simulink model "ModelAgriAuto"  (R2022a)
settings: Solver=FixedStepAuto  StartTime=0.0  StopTime=6240  FixedStep=0.05  MaxStep=0.1  RelTol=1e-3
model workspace (MAT data in the model file):
  PlowHectare = 1.925
values from neighbouring files (symbols this model uses):
  C_rate = 3    [start_function.m]
  Compaction = 0    [start_function.m]
  CyclesIn = CyclesIn+CyclesOut(end)    [start_function.m]
  Degradation = 2    [start_function.m]
  FailRate = 29700000    [start_function.m]
  FieldEff = 0.8    [start_function.m]
  ForceCorrVar = 0.85    [start_function.m]
  Fuel = 3    [start_function.m]
  Mass = 10550    [start_function.m]
  n = n+1    (= 2)    [start_function.m]
  v_field = 5    [start_function.m]
  Weather_crit = 3    [start_function.m]
  WorkingHours = 10    [start_function.m]
undefined symbols (not defined in the file or in its folder): Battery, BatteryNo, Charger, ChargerNo, DField, m, Power, Soil, TractorNo, Year
libraries: simulink x2
(part 2 of 3)

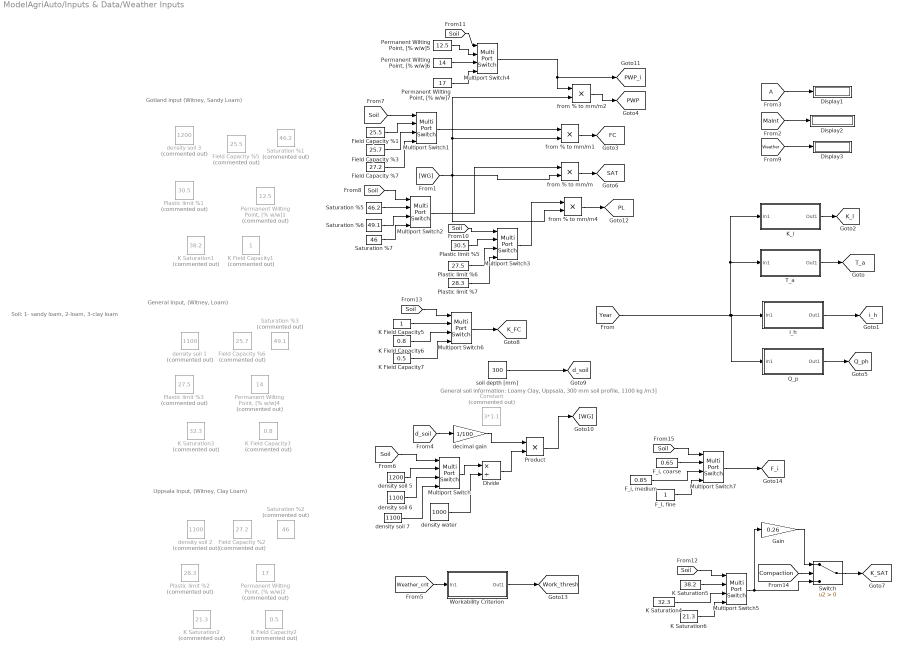
== system ModelAgriAuto/Inputs & Data/Weather Inputs ==
  note: Soil: 1- sandy loam, 2-loam, 3-clay loam
  note: Uppsala Input, (Witney, Clay Loam)
  note: Gotland input (Witney, Sandy Loam)
  note: General soil information: Loamy Clay, Uppsala, 300 mm soil profile, 1100 kg /m3]
  note: General Input, (Witney, Loam)
  Constant : Constant  Commented=on  Value=3*1.1
  Display1 : Display
  Display2 : Display
  Display3 : Display
  Divide : Product  Inputs=*/
  "F_I, fine" : Constant
  "F_i, coarse" : Constant  Value=0.65
  "F_i, medium" : Constant  Value=0.85
  Field Capacity %1 : Constant  Value=25.5
  Field Capacity %2 : Constant  Commented=on  Value=27.2
  Field Capacity %3 : Constant  Value=25.7
  Field Capacity %5 : Constant  Commented=on  Value=25.5
  Field Capacity %6 : Constant  Commented=on  Value=25.7
  Field Capacity %7 : Constant  Value=27.2
  From3 : From  TagVisibility=global
  Gain : Gain  Gain=0.26
  K Field Capacity1 : Constant  Commented=on
  K Field Capacity2 : Constant  Commented=on  Value=0.5
  K Field Capacity3 : Constant  Commented=on  Value=0.8
  K Field Capacity5 : Constant
  K Field Capacity6 : Constant  Value=0.8
  K Field Capacity7 : Constant  Value=0.5
  K Saturation1 : Constant  Commented=on  Value=38.2
  K Saturation2 : Constant  Commented=on  Value=21.3
  K Saturation3 : Constant  Commented=on  Value=32.3
  K Saturation4 : Constant  Value=32.3
  K Saturation5 : Constant  Value=38.2
  K Saturation6 : Constant  Value=21.3
  K_l : Subsystem
  Multiport Switch{,1..7} (8 alike) : MultiPortSwitch  SaturateOnIntegerOverflow=off  InputSameDT=off
  "Permanent Wilting Point, [% w/w]1" : Constant  Commented=on  Value=12.5
  "Permanent Wilting Point, [% w/w]2" : Constant  Commented=on  Value=17
  "Permanent Wilting Point, [% w/w]4" : Constant  Commented=on  Value=14
  "Permanent Wilting Point, [% w/w]5" : Constant  Value=12.5
  "Permanent Wilting Point, [% w/w]6" : Constant  Value=14
  "Permanent Wilting Point, [% w/w]7" : Constant  Value=17
  Plastic limit %1 : Constant  Commented=on  Value=30.5
  Plastic limit %2 : Constant  Commented=on  Value=28.3
  Plastic limit %3 : Constant  Commented=on  Value=27.5
  Plastic limit %5 : Constant  Value=30.5
  Plastic limit %6 : Constant  Value=27.5
  Plastic limit %7 : Constant  Value=28.3
  Product : Product
  Q_p : Subsystem
  Saturation %1 : Constant  Commented=on  Value=46.2
  Saturation %2 : Constant  Commented=on  Value=46
  Saturation %3 : Constant  Commented=on  Value=49.1
  Saturation %5 : Constant  Value=46.2
  Saturation %6 : Constant  Value=49.1
  Saturation %7 : Constant  Value=46
  Switch : Switch  Criteria=u2 > Threshold  SaturateOnIntegerOverflow=off  InputSameDT=off
  T_a : Subsystem
  "Workability Criterion " : Subsystem
  decimal gain : Gain  Gain=1/100
  density soil 1 : Constant  Commented=on  Value=1100
  density soil 2 : Constant  Commented=on  Value=1100
  density soil 3 : Constant  Commented=on  Value=1200
  density soil 5 : Constant  Value=1200
  density soil 6 : Constant  Value=1100
  density soil 7 : Constant  Value=1100
  "density water " : Constant  Value=1000
  from % to mm/m{,1..2,4} (4 alike) : Product
  i_h : Subsystem
  soil depth [mm] : Constant  Value=300
  tag scope: FC=global, F_i=global, K_FC=global, K_SAT=global, K_l=global, PL=global, PWP=global, PWP_i=global, Q_ph=global, SAT=global, T_a=global, Work_thresh=global, d_soil=global, i_h=global
  wires:
  K_l/1(Out1) -> [K_l]
  T_a/1(Out1) -> [T_a]
  i_h/1(Out1) -> [i_h]
  Q_p/1(Out1) -> [Q_ph]
  From3/1 -> Display1/1
  [Weather] -> Display3/1
  [MaInt] -> Display2/1
  Multiport Switch4/1 -> from % to mm/m2/1, [PWP_i]
  Multiport Switch2/1 -> from % to mm/m/1
  Multiport Switch6/1 -> [K_FC]
  soil depth [mm]/1 -> [d_soil]
  [WG] -> from % to mm/m4/2, from % to mm/m2/2, from % to mm/m1/2, from % to mm/m/2
  from % to mm/m/1 -> [SAT]
  from % to mm/m1/1 -> [FC]
  from % to mm/m2/1 -> [PWP]
  Divide/1 -> Product/2
  [d_soil] -> decimal gain/1
  "density water "/1 -> Divide/2
  decimal gain/1 -> Product/1
  Product/1 -> [WG]
  Multiport Switch3/1 -> from % to mm/m4/1
  from % to mm/m4/1 -> [PL]
  Multiport Switch/1 -> Divide/1
  Multiport Switch1/1 -> from % to mm/m1/1
  [Soil] -> Multiport Switch/1
  density soil 5/1 -> Multiport Switch/2
  density soil 6/1 -> Multiport Switch/3
  density soil 7/1 -> Multiport Switch/4
  [Soil] -> Multiport Switch1/1
  Field Capacity %7/1 -> Multiport Switch1/4
  Field Capacity %1/1 -> Multiport Switch1/2
  Field Capacity %3/1 -> Multiport Switch1/3
  Saturation %7/1 -> Multiport Switch2/4
  [Soil] -> Multiport Switch2/1
  Saturation %5/1 -> Multiport Switch2/2
  Saturation %6/1 -> Multiport Switch2/3
  [Soil] -> Multiport Switch3/1
  Plastic limit %5/1 -> Multiport Switch3/2
  Plastic limit %6/1 -> Multiport Switch3/3
  Plastic limit %7/1 -> Multiport Switch3/4
  "Workability Criterion "/1(Out1) -> [Work_thresh]
  [Weather_crit] -> "Workability Criterion "/1(In1)
  "Permanent Wilting Point, [% w/w]6"/1 -> Multiport Switch4/3
  [Soil] -> Multiport Switch4/1
  "Permanent Wilting Point, [% w/w]5"/1 -> Multiport Switch4/2
  "Permanent Wilting Point, [% w/w]7"/1 -> Multiport Switch4/4
  K Saturation4/1 -> Multiport Switch5/3
  [Soil] -> Multiport Switch5/1
  K Saturation6/1 -> Multiport Switch5/4
  K Saturation5/1 -> Multiport Switch5/2
  K Field Capacity7/1 -> Multiport Switch6/4
  [Soil] -> Multiport Switch6/1
  K Field Capacity5/1 -> Multiport Switch6/2
  K Field Capacity6/1 -> Multiport Switch6/3
  [Compaction] -> Switch/2
  Multiport Switch5/1 -> Gain/1, Switch/3
  Switch/1 -> [K_SAT]
  Gain/1 -> Switch/1
  "F_I, fine"/1 -> Multiport Switch7/4
  "F_i, medium"/1 -> Multiport Switch7/3
  "F_i, coarse"/1 -> Multiport Switch7/2
  [Soil] -> Multiport Switch7/1
  Multiport Switch7/1 -> [F_i]
  [Year] -> K_l/1(In1), T_a/1(In1), Q_p/1(In1), i_h/1(In1)

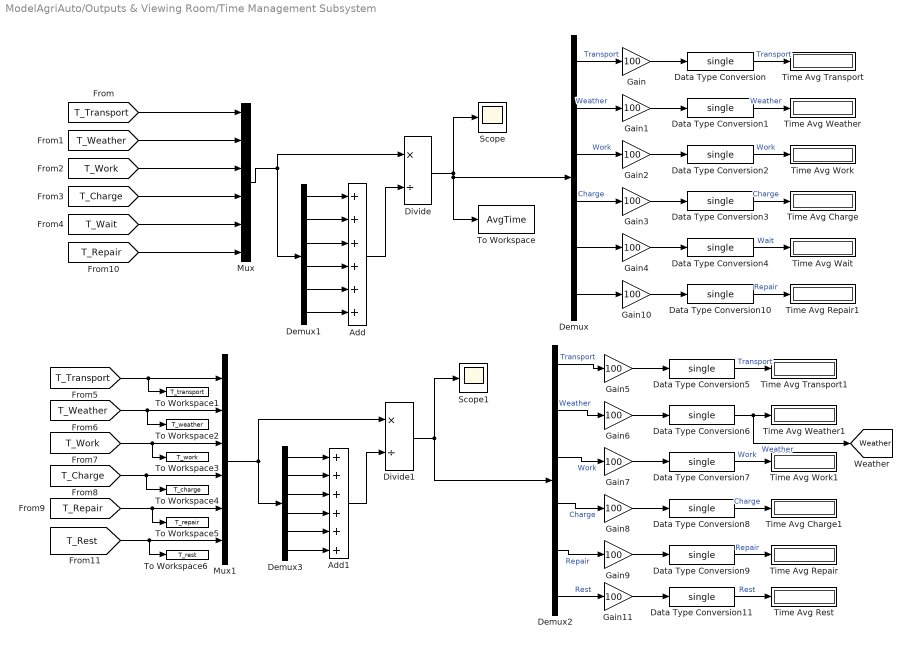
== system ModelAgriAuto/Outputs & Viewing Room/Time Management Subsystem ==
  Add : Sum  Inputs=++++++
  Add1 : Sum  Inputs=++++++
  Data Type Conversion{,1..11} (12 alike) : DataTypeConversion  OutDataTypeStr=single  SaturateOnIntegerOverflow=off  RndMeth=Floor
  Demux{,1..3} (4 alike) : Demux  Outputs=6
  Divide : Product  Inputs=*/
  Divide1 : Product  Inputs=*/
  Gain{,1..11} (12 alike) : Gain  Gain=100
  Mux : Mux  Inputs=6
  Mux1 : Mux  Inputs=6
  Scope : Scope
  Scope1 : Scope
  Time Avg Charge : Display
  Time Avg Charge1 : Display
  Time Avg Repair : Display
  Time Avg Repair1 : Display
  Time Avg Rest : Display
  Time Avg Transport : Display
  Time Avg Transport1 : Display
  Time Avg Wait : Display
  Time Avg Weather : Display
  Time Avg Weather1 : Display
  Time Avg Work : Display
  Time Avg Work1 : Display
  To Workspace : ToWorkspace  VariableName=AvgTime  SaveFormat=Timeseries  SampleTime=1
  To Workspace1 : ToWorkspace  VariableName=T_transport  SampleTime=1
      settings: Save2DSignal=2-D array (concatenate along first dimension)
  To Workspace2 : ToWorkspace  VariableName=T_weather  SampleTime=1
      settings: Save2DSignal=2-D array (concatenate along first dimension)
  To Workspace3 : ToWorkspace  VariableName=T_work  SampleTime=1
      settings: Save2DSignal=2-D array (concatenate along first dimension)
  To Workspace4 : ToWorkspace  VariableName=T_charge  SampleTime=1
      settings: Save2DSignal=2-D array (concatenate along first dimension)
  To Workspace5 : ToWorkspace  VariableName=T_repair  SampleTime=1
      settings: Save2DSignal=2-D array (concatenate along first dimension)
  To Workspace6 : ToWorkspace  VariableName=T_rest  SampleTime=1
      settings: Save2DSignal=2-D array (concatenate along first dimension)
  tag scope: Weather=global
  wires:
  [T_Transport] -> Mux/1
  [T_Weather] -> Mux/2
  [T_Work] -> Mux/3
  [T_Charge] -> Mux/4
  Mux/1 -> Divide/1, Demux1/1
  Divide/1 -> Demux/1, To Workspace/1, Scope/1
  Demux/1 -> Gain/1  "Transport"
  Demux/2 -> Gain1/1  "Weather"
  Demux/3 -> Gain2/1  "Work"
  Demux/4 -> Gain3/1  "Charge"
  Demux1/2 -> Add/2
  Demux1/1 -> Add/1
  Demux1/3 -> Add/3
  Demux1/4 -> Add/4
  Add/1 -> Divide/2
  Data Type Conversion/1 -> Time Avg Transport/1  "Transport"
  Data Type Conversion1/1 -> Time Avg Weather/1  "Weather"
  Data Type Conversion2/1 -> Time Avg Work/1  "Work"
  Data Type Conversion3/1 -> Time Avg Charge/1  "Charge"
  Gain/1 -> Data Type Conversion/1
  Gain1/1 -> Data Type Conversion1/1
  Gain2/1 -> Data Type Conversion2/1
  Gain3/1 -> Data Type Conversion3/1
  [T_Wait] -> Mux/5
  Demux1/5 -> Add/5
  Demux/5 -> Gain4/1
  Gain4/1 -> Data Type Conversion4/1
  Data Type Conversion4/1 -> Time Avg Wait/1  "Wait"
  Data Type Conversion5/1 -> Time Avg Transport1/1  "Transport"
  Mux1/1 -> Divide1/1, Demux3/1
  Demux2/3 -> Gain7/1  "Work"
  Demux2/1 -> Gain5/1  "Transport"
  [T_Charge] -> To Workspace4/1, Mux1/4
  Demux3/4 -> Add1/4
  Add1/1 -> Divide1/2
  Gain6/1 -> Data Type Conversion6/1
  Demux3/3 -> Add1/3
  Gain5/1 -> Data Type Conversion5/1
  [T_Work] -> To Workspace3/1, Mux1/3
  Demux2/4 -> Gain8/1  "Charge"
  [T_Transport] -> To Workspace1/1, Mux1/1
  Gain8/1 -> Data Type Conversion8/1
  Gain7/1 -> Data Type Conversion7/1
  Divide1/1 -> Scope1/1, Demux2/1
  Data Type Conversion6/1 -> [Weather], Time Avg Weather1/1  "Weather"
  [T_Weather] -> To Workspace2/1, Mux1/2
  Demux3/1 -> Add1/1
  Data Type Conversion7/1 -> Time Avg Work1/1  "Work"
  Data Type Conversion8/1 -> Time Avg Charge1/1  "Charge"
  Demux2/2 -> Gain6/1  "Weather"
  Demux3/2 -> Add1/2
  [T_Repair] -> To Workspace5/1, Mux1/5
  Demux3/5 -> Add1/5
  Demux2/5 -> Gain9/1  "Repair"
  Gain9/1 -> Data Type Conversion9/1
  Data Type Conversion9/1 -> Time Avg Repair/1  "Repair"
  [T_Repair] -> Mux/6
  Demux1/6 -> Add/6
  Gain10/1 -> Data Type Conversion10/1
  Data Type Conversion10/1 -> Time Avg Repair1/1  "Repair"
  Demux/6 -> Gain10/1
  [T_Rest] -> To Workspace6/1, Mux1/6
  Demux3/6 -> Add1/6
  Gain11/1 -> Data Type Conversion11/1
  Data Type Conversion11/1 -> Time Avg Rest/1  "Rest"
  Demux2/6 -> Gain11/1  "Rest"

== system ModelAgriAuto/Time & Weather subsyst./Driver work-time subsystem ==
  note: Working time check
  In1 : Inport
  Add : Sum  Inputs=+-
  Avg wait time [h]1 : Display
  Constant : Constant  Value=0
  Constant1 : Constant
  Counter Limited : simulink/Sources/Counter Limited  uplimit=24  tsamp=1
  Entity Gate : EntityGate  InputPortMessageModes=m,m  OutputPortMessageModes=m  OpenGateAtSimulationStart=on
  Entity Queue2 : Queue  InputPortMessageModes=m  OutputPortMessageModes=n,n,m  NumberEntitiesDeparted=on  AverageWait=on
      settings: OutputPortMap=o0,o2,o5
  Message Send1 : Send  OutputPortMessageModes=m
  Product : Product
  Switch : Switch  SaturateOnIntegerOverflow=off  InputSameDT=off
  Out1 : Outport
  tag scope: T_Rest=global
  wires:
  Add/1 -> Switch/2
  [WorkingHours] -> Add/2
  Constant/1 -> Switch/1
  Constant1/1 -> Switch/3
  Counter Limited/1 -> Add/1
  In1/1 -> Entity Queue2/1
  Entity Queue2/3 -> Entity Gate/2
  Entity Gate/1 -> Out1/1
  Message Send1/1 -> Entity Gate/1
  Switch/1 -> Message Send1/1
  Entity Queue2/1 -> Product/2
  Entity Queue2/2 -> Product/1
  Product/1 -> Avg wait time [h]1/1, [T_Rest]

== system ModelAgriAuto/Time & Weather subsyst./Weather & schedule subsystem ==
  note: From Alfredo (2004)
  note: Working time check
  note: Soil moisture check
  In1 : Inport
  % of days workable : Display
  Add : Sum  Inputs=+-
  Avg wait time [h]1 : Display
  Clock1 : Clock
  Constant : Constant  Value=0
  Constant1 : Constant
  Counter Limited : simulink/Sources/Counter Limited  uplimit=24  tsamp=1
  "Daily soil water content model " : Subsystem
  Divide1 : Product  Inputs=*/
  Entity Gate : EntityGate  InputPortMessageModes=m,m  OutputPortMessageModes=m  OpenGateAtSimulationStart=on
  Entity Queue2 : Queue  InputPortMessageModes=m  OutputPortMessageModes=n,n,m  NumberEntitiesDeparted=on  AverageWait=on
      settings: OutputPortMap=o0,o2,o5
  Gain : Gain  Gain=100
  Integrator : Integrator
  Integrator1 : Integrator
  Message Send1 : Send  OutputPortMessageModes=m
  Product : Product
  Product1 : Product
  Relational Operator1 : RelationalOperator  Operator=<=  OutDataTypeStr='double'  InputSameDT=off
  Scope : Scope
  Scope1 : Scope  NumInputPorts=2
  Switch : Switch  SaturateOnIntegerOverflow=off  InputSameDT=off
  Threshold value (mm/m) : Display
  To Workspace : ToWorkspace  VariableName=WeatherWaitTime1  SaveFormat=Timeseries  SampleTime=1
  To Workspace1 : ToWorkspace  VariableName=m_a1  SampleTime=1
  Utilization : Scope
  Workable : Goto  TagVisibility=global
  Out1 : Outport  VectorParamsAs1DForOutWhenUnconnected=off
  tag scope: MaInt=global, T_Weather=global, Workability=global
  wires:
  Entity Queue2/3 -> Entity Gate/2
  Clock1/1 -> Divide1/2
  [Work_thresh] -> Relational Operator1/2, Threshold value (mm/m)/1
  Entity Gate/1 -> Out1/1
  Entity Queue2/1 -> Product/2
  Divide1/1 -> Workable/1, Gain/1
  Relational Operator1/1 -> Scope1/1, Product1/1, [Workability], Utilization/1, Integrator1/1
  Gain/1 -> % of days workable/1
  Switch/1 -> Scope1/2, Product1/2
  Message Send1/1 -> Entity Gate/1
  Entity Queue2/2 -> Avg wait time [h]1/1, Product/1
  Integrator/1 -> [MaInt]
  Integrator1/1 -> Divide1/1
  Add/1 -> Switch/2
  [WorkingHours] -> Add/2
  "Daily soil water content model "/1(m_a (Soil moisture content [mm/m])) -> Integrator/1, To Workspace1/1, Relational Operator1/1
  In1/1 -> Entity Queue2/1
  Constant/1 -> Switch/1
  Product1/1 -> Scope/1, Message Send1/1
  Constant1/1 -> Switch/3
  Counter Limited/1 -> Add/1
  Product/1 -> [T_Weather], To Workspace/1

== system ModelAgriAuto/Transport Subsystem/Road forces ==
  "m " : Inport
  a : Inport  Port=2
  "N_block " : Inport  Port=3
  *g : Gain  Gain=9.81
  Crr_road : Constant  Value=0.1
  Display : Display
  Drag force road : MATLAB Function  TreatAsAtomicUnit=on
  Integrator : Integrator
  "Net force needed [N] " : Sum
  P [kW] : Scope
  "P [kW] " : Product  Inputs=3
  "Rolling resistance road " : Product
  Scope : Scope
  Subsystem : Subsystem
  "W to kW " : Constant  Value=0.001
  kWs to kWh : Gain  Gain=1/3600
  km/h to m/s : Gain  Gain=1/3.6
  tag scope: F_road=global, P_road=global, v_road=global
  wires:
  [v_road_actual] -> km/h to m/s/1, Drag force road/1(v)
  Drag force road/1(F_drag_road) -> "Net force needed [N] "/2
  a/1 -> Subsystem/1(a)
  "m "/1 -> *g/1
  Crr_road/1 -> "Rolling resistance road "/1
  *g/1 -> "Rolling resistance road "/2
  "Rolling resistance road "/1 -> "Net force needed [N] "/1
  "Net force needed [N] "/1 -> [F_road], "P [kW] "/1
  "W to kW "/1 -> "P [kW] "/3
  km/h to m/s/1 -> [v_road], "P [kW] "/2
  kWs to kWh/1 -> Scope/1
  "P [kW] "/1 -> Integrator/1, Display/1, [P_road], P [kW]/1
  Integrator/1 -> kWs to kWh/1
  "N_block "/1 -> Subsystem/2(In1)

== system ModelAgriAuto/Inputs & Data/Battery and driveline inputs/Battery capacity reduction ==
  Add : Sum  Inputs=++++
  Add1 : Sum
  Add2 : Sum
  Charging rate choice : Subsystem
  Constant4 : Constant  Value=BatteryNo
  Constant5 : Constant  Value=CyclesIn
  Constant7 : Constant  Value=TractorNo
  Constant8 : Constant  Value=0
  Display : Display
  Display1 : Display
  Display2 : Display
  Divide : Product  Inputs=*/
  Memory : Memory  InitialCondition=CyclesIn
  Product1 : Product  Inputs=3
  Product2 : Product
  Product4 : Product  Inputs=4
  Saturation : Saturate  UpperLimit=1
  Scope : Scope
  Switch : Switch  Criteria=u2 > Threshold  Threshold=1  SaturateOnIntegerOverflow=off  InputSameDT=off
  To Workspace : ToWorkspace  VariableName=CyclesOut  SampleTime=-1
      settings: Save2DSignal=2-D array (concatenate along first dimension)
  Out1 : Outport  VectorParamsAs1DForOutWhenUnconnected=off
  wires:
  Product1/1 -> Add/2
  Product2/1 -> Add/3
  Add/1 -> Saturation/1
  [Charge_no] -> Display1/1, Divide/1
  Saturation/1 -> Display2/1, Scope/1, Out1/1
  Product4/1 -> Add/1
  Memory/1 -> Display/1, Product4/4, Product4/2, Product4/3, Product1/2, Product1/3, Product2/1
  Constant4/1 -> Switch/1
  Divide/1 -> To Workspace/1, Add1/1
  Constant5/1 -> Add1/2
  Add1/1 -> Memory/1
  Constant7/1 -> Add2/2
  Add2/1 -> Divide/2
  Constant8/1 -> Switch/3
  Switch/1 -> Add2/1
  [Fuel] -> Switch/2
  Charging rate choice/1(Out1) -> Product4/1
  Charging rate choice/2(Out2) -> Product1/1
  Charging rate choice/3(Out3) -> Product2/2
  Charging rate choice/4(Out4) -> Add/4

== system ModelAgriAuto/Inputs & Data/Field inputs/Field efficiancy ==
  note: 0.8 From Witney
  Crop choice : MultiPortSwitch  Commented=on  Inputs=12  SaturateOnIntegerOverflow=off  InputSameDT=off
  Demux1 : Demux  Commented=on  Outputs=12
  Field effiency : Constant  Commented=on  Value=0.8  SampleTime=100000
  Field sizes [ha]1 : Constant  Commented=on  Value=[0.8 0.8 0.8 0.8 0.8 0.8 0.8 0.8 0.8 0.8 0.8 0.8]
  From2 : From  Commented=on  GotoTag=Field  TagVisibility=global
  Goto1 : Goto  Commented=on  GotoTag=field_eff  TagVisibility=global
  Goto4 : Goto  Commented=on  GotoTag=field_eff  TagVisibility=global
  wires:
  Field effiency/1 -> Goto4/1
  From2/1 -> Crop choice/1
  Demux1/5 -> Crop choice/6
  Demux1/6 -> Crop choice/7
  Demux1/9 -> Crop choice/10
  Demux1/7 -> Crop choice/8
  Demux1/3 -> Crop choice/4
  Demux1/2 -> Crop choice/3
  Demux1/8 -> Crop choice/9
  Demux1/12 -> Crop choice/13
  Demux1/4 -> Crop choice/5
  Demux1/10 -> Crop choice/11
  Demux1/11 -> Crop choice/12
  Demux1/1 -> Crop choice/2
  Field sizes [ha]1/1 -> Demux1/1
  Crop choice/1 -> Goto1/1

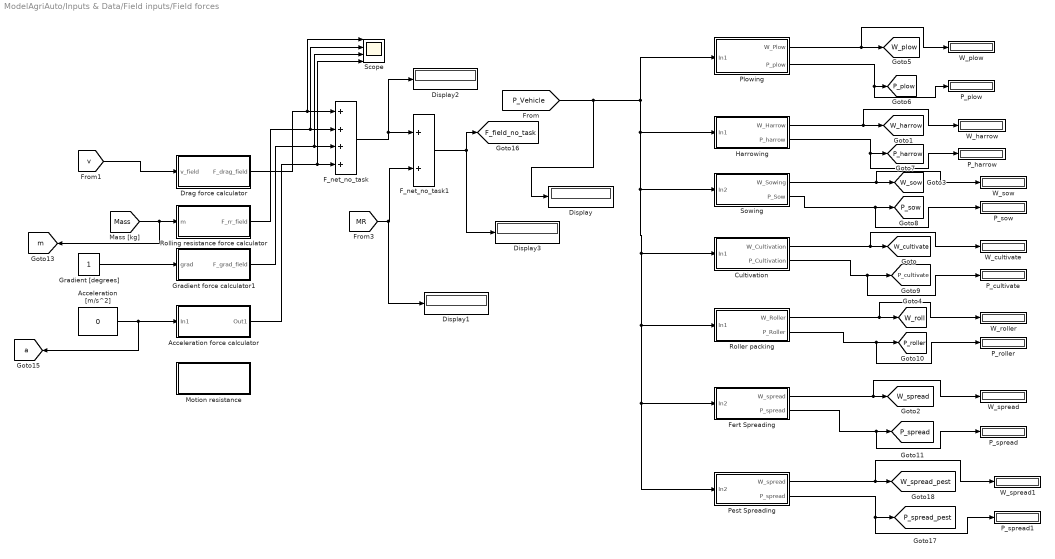
== system ModelAgriAuto/Inputs & Data/Field inputs/Field forces ==
  Acceleration [m/s^2] : Constant  Value=0
  Acceleration force calculator : Subsystem
  Cultivation : Subsystem
  Display{,1..3} (4 alike) : Display
  Drag force calculator : Subsystem
  F_net_no_task : Sum  Inputs=4
  F_net_no_task1 : Sum  Inputs=2
  Fert Spreading : Subsystem
  Gradient [degrees] : Constant
  Gradient force calculator1 : Subsystem
  Harrowing : Subsystem
  "Motion resistance " : Subsystem
  P_cultivate : Display
  P_harrow : Display
  P_plow : Display
  P_roller : Display
  P_sow : Display
  P_spread : Display
  P_spread1 : Display
  Pest Spreading : Subsystem
  Plowing : Subsystem
  Roller packing : Subsystem
  Rolling resistance force calculator : Subsystem
  Scope : Scope  NumInputPorts=4
  Sowing : Subsystem
  W_cultivate : Display
  W_harrow : Display
  W_plow : Display
  W_roller : Display
  W_sow : Display
  W_spread : Display
  W_spread1 : Display
  tag scope: F_field_no_task=global, P_cultivate=global, P_harrow=global, P_plow=global, P_roller=global, P_sow=global, P_spread=global, P_spread_pest=global, W_cultivate=global, W_harrow=global, W_plow=global, W_roll=global, W_sow=global, W_spread=global, W_spread_pest=global, a=global, m=global
  wires:
  Cultivation/1(W_Cultivation) -> W_cultivate/1, [W_cultivate]
  Roller packing/1(W_Roller) -> W_roller/1, [W_roll]
  Plowing/1(W_Plow) -> W_plow/1, [W_plow]
  Sowing/1(W_Sowing) -> W_sow/1, [W_sow]
  Harrowing/1(W_Harrow) -> W_harrow/1, [W_harrow]
  [P_Vehicle] -> Display/1, Sowing/1(In2), Cultivation/1(In1), Pest Spreading/1(In2), Fert Spreading/1(In2), Roller packing/1(In1), Harrowing/1(In1), Plowing/1(In1)
  Fert Spreading/1(W_spread) -> W_spread/1, [W_spread]
  Plowing/2(P_plow) -> P_plow/1, [P_plow]
  Harrowing/2(P_harrow) -> P_harrow/1, [P_harrow]
  Sowing/2(P_Sow) -> P_sow/1, [P_sow]
  Cultivation/2(P_Cultivation) -> P_cultivate/1, [P_cultivate]
  Roller packing/2(P_Roller) -> P_roller/1, [P_roller]
  Fert Spreading/2(P_spread) -> P_spread/1, [P_spread]
  F_net_no_task1/1 -> Display3/1, [F_field_no_task]
  [Mass] -> Rolling resistance force calculator/1(m), [m]
  Gradient [degrees]/1 -> Gradient force calculator1/1(grad)
  Rolling resistance force calculator/1(F_rr_field) -> Scope/2, F_net_no_task/2
  Acceleration force calculator/1(Out1) -> Scope/4, F_net_no_task/4
  Acceleration [m/s^2]/1 -> [a], Acceleration force calculator/1(In1)
  Drag force calculator/1(F_drag_field) -> Scope/1, F_net_no_task/1
  Pest Spreading/2(P_spread) -> P_spread1/1, [P_spread_pest]
  Pest Spreading/1(W_spread) -> W_spread1/1, [W_spread_pest]
  F_net_no_task/1 -> Display2/1, F_net_no_task1/1
  [MR] -> Display1/1, F_net_no_task1/2
  Gradient force calculator1/1(F_grad_field) -> Scope/3, F_net_no_task/3
  [v] -> Drag force calculator/1(v_field)

== system ModelAgriAuto/Inputs & Data/Field inputs/Fieldwork choice & data ==
  Crop choice : MultiPortSwitch  Inputs=12  SaturateOnIntegerOverflow=off  InputSameDT=off
  Demux : Demux  Outputs=16
  Demux1 : Demux  Outputs=12
  Fall period no. tasks : Constant  Value=8
  Havre / Oats : Subsystem
  Höstvete / Winter Wheat : Subsystem
  Korn / Barley : Subsystem
  Multiport Switch : MultiPortSwitch  Inputs=4  SaturateOnIntegerOverflow=off  InputSameDT=off
  Spring period no. tasks : Constant  Value=5
  Subsystem : Subsystem
  "Summer period no. tasks " : Constant  Value=3
  Task : MultiPortSwitch  Inputs=16  DiagnosticForDefault=None  SaturateOnIntegerOverflow=off  InputSameDT=off
  To Workspace : ToWorkspace  VariableName=P_vehicle  SampleTime=1
  To Workspace1 : ToWorkspace  VariableName=P_task  SampleTime=1
  To Workspace2 : ToWorkspace  VariableName=Task_no  SampleTime=1
  Vårvete / Spring wheat : Subsystem
  tag scope: P_fieldwork=global, W_fieldwork=global, X_1=global, X_2=global, X_3=global, X_val=global
  wires:
  Korn / Barley/1(Barley) -> Multiport Switch/3
  Havre / Oats/1(Oats) -> Multiport Switch/2
  Vårvete / Spring wheat/1(Spring Wheat) -> Multiport Switch/4
  Höstvete / Winter Wheat/1(Winter Wheat) -> Multiport Switch/5
  Subsystem/1(P) -> To Workspace1/1, [P_fieldwork]
  Subsystem/2(W) -> [W_fieldwork]
  Demux1/1 -> Crop choice/2
  Demux1/10 -> Crop choice/11
  Demux1/12 -> Crop choice/13
  Demux1/2 -> Crop choice/3
  Demux1/4 -> Crop choice/5
  Demux1/6 -> Crop choice/7
  [Rotation_choice] -> Demux1/1
  Demux1/11 -> Crop choice/12
  Demux1/3 -> Crop choice/4
  Demux1/9 -> Crop choice/10
  Demux1/7 -> Crop choice/8
  Demux1/8 -> Crop choice/9
  Demux1/5 -> Crop choice/6
  [Field] -> Crop choice/1
  Crop choice/1 -> Multiport Switch/1
  Spring period no. tasks/1 -> [X_1]
  "Summer period no. tasks "/1 -> [X_2]
  Fall period no. tasks/1 -> [X_3]
  Multiport Switch/1 -> Demux/1
  Task/1 -> [X_val], Subsystem/1(In1)
  Demux/1 -> Task/2
  Demux/2 -> Task/3
  Demux/3 -> Task/4
  Demux/4 -> Task/5
  Demux/5 -> Task/6
  Demux/6 -> Task/7
  Demux/7 -> Task/8
  Demux/8 -> Task/9
  Demux/9 -> Task/10
  Demux/10 -> Task/11
  Demux/11 -> Task/12
  Demux/12 -> Task/13
  Demux/13 -> Task/14
  Demux/14 -> Task/15
  Demux/15 -> Task/16
  Demux/16 -> Task/17
  [X] -> To Workspace2/1, Task/1
  [P_no_task] -> To Workspace/1

== system ModelAgriAuto/Inputs & Data/Weather Inputs/K_l ==
  In1 : Inport
  K_I Average (used for 2007-1989) : Constant  Value=|
      | [0.450028847727057
      | 0.607359298852742
      | 0.765426053964252
      | 0.7333871392247
      | 0.753122156456283
      | 0.621245449686598
      | 0.471386923430517
      | 0.305528183242989]
  K_i Gotland 2016 : Constant  Value="[0.324387225 0.562819073\t0.660046574 0.6480848 0.651225532 0.554589293 0.574529657 0.209079905]"
  K_l 2008 : Constant  Value=|
      | [0.374226548964607
      | 0.5651112088906
      | 0.846502244344832
      | 0.857597160728091
      | 0.887293097073643
      | 0.407509006407612
      | 0.309263537111899
      | 0.304514356779021]
  K_l 2009 : Constant  Value=|
      | [0.262637998942759
      | 0.771519126584715
      | 0.792961099041455
      | 0.72258278408761
      | 0.606394778575292
      | 0.716095726119652
      | 0.589821155203549
      | 0.285040196536773]
  K_l 2010 : Constant  Value=|
      | [0.452397430843929
      | 0.551642848194288
      | 0.679396333880287
      | 0.897808211643704
      | 0.830797941741758
      | 0.473775235511066
      | 0.446647538554147
      | 0.356666727778847]
  K_l 2011 : Constant  Value=|
      | [0.587965636620863
      | 0.689844225051716
      | 0.78618604992254
      | 0.900157211084527
      | 0.635451328731586
      | 0.581509134743191
      | 0.47043316313591
      | 0.396692150445966]
  K_l 2012 : Constant  Value=|
      | [0.492566467135397
      | 0.503980694662157
      | 0.859577959280954
      | 0.570282827171698
      | 0.681327478786434
      | 0.562646860208943
      | 0.402221274983423
      | 0.236984633342195]
  K_l 2013 : Constant  Value=|
      | [0.704879349277501
      | 0.650358117378165
      | 0.784679634671385
      | 0.725744575530072
      | 0.805986396428604
      | 0.747398912814307
      | 0.5288709219078
      | 0.3126422767954]
  K_l 2014 : Constant  Value=|
      | [0.45160373639872
      | 0.703059734100902
      | 0.606012827446703
      | 0.571640281482704
      | 0.926149749287279
      | 0.637762133059551
      | 0.669181432897298
      | 0.141948317428888]
  K_l 2015 : Constant  Value=|
      | [0.436590765338393
      | 0.633648519404645
      | 0.588557660870176
      | 0.679524669459493
      | 0.583771049326697
      | 0.935386091478823
      | 0.458611011803818
      | 0.440120757668815]
  K_l 2016 : Constant  Value=|
      | [0.324646236864701
      | 0.509461693357412
      | 0.82927854015223
      | 0.808272755884339
      | 0.862643499039011
      | 0.576023552634393
      | 0.56627539593054
      | 0.241738397088616]
  K_l 2017 : Constant  Value=|
      | [0.407514353723412
      | 0.572464532018199
      | 0.845299862192033
      | 0.767298566613805
      | 0.769110542767832
      | 0.658206449168416
      | 0.274764947275466
      | 0.247055156798577]
  K_l 2018 : Constant  Value=|
      | [0.455288801
      | 0.529861588
      | 0.801234382
      | 0.566349488
      | 0.695417859
      | 0.537386844
      | 0.469165779
      | 0.397407045]
  Multiport Switch3 : MultiPortSwitch  Inputs=31  SaturateOnIntegerOverflow=off  InputSameDT=off
  Out1 : Outport  VectorParamsAs1DForOutWhenUnconnected=off
  wires:
  Multiport Switch3/1 -> Out1/1
  In1/1 -> Multiport Switch3/1
  K_I Average (used for 2007-1989)/1 -> Multiport Switch3/6, Multiport Switch3/7, Multiport Switch3/8, Multiport Switch3/9, Multiport Switch3/10, Multiport Switch3/11, Multiport Switch3/12, Multiport Switch3/13, Multiport Switch3/14, Multiport Switch3/20, Multiport Switch3/19, Multiport Switch3/15, Multiport Switch3/16, Multiport Switch3/18, Multiport Switch3/17, Multiport Switch3/2, Multiport Switch3/3, Multiport Switch3/4, Multiport Switch3/5
  K_l 2008/1 -> Multiport Switch3/21
  K_l 2009/1 -> Multiport Switch3/22
  K_l 2010/1 -> Multiport Switch3/23
  K_l 2011/1 -> Multiport Switch3/24
  K_l 2012/1 -> Multiport Switch3/25
  K_l 2014/1 -> Multiport Switch3/27
  K_l 2016/1 -> Multiport Switch3/29
  K_l 2013/1 -> Multiport Switch3/26
  K_l 2015/1 -> Multiport Switch3/28
  K_l 2017/1 -> Multiport Switch3/30
  K_l 2018/1 -> Multiport Switch3/31
  K_i Gotland 2016/1 -> Multiport Switch3/32

== system ModelAgriAuto/Inputs & Data/Weather Inputs/Q_p ==
  In1 : Inport
  Demux : Demux  Outputs=31
  From Workspace : FromWorkspace  VariableName=Q_pTable
  Multiport Switch1 : MultiPortSwitch  Inputs=31  SaturateOnIntegerOverflow=off  InputSameDT=off
  Out1 : Outport  VectorParamsAs1DForOutWhenUnconnected=off
  wires:
  In1/1 -> Multiport Switch1/1
  Multiport Switch1/1 -> Out1/1
  Demux/1 -> Multiport Switch1/2
  Demux/2 -> Multiport Switch1/3
  Demux/3 -> Multiport Switch1/4
  Demux/4 -> Multiport Switch1/5
  Demux/5 -> Multiport Switch1/6
  Demux/6 -> Multiport Switch1/7
  Demux/7 -> Multiport Switch1/8
  Demux/8 -> Multiport Switch1/9
  Demux/9 -> Multiport Switch1/10
  Demux/10 -> Multiport Switch1/11
  Demux/11 -> Multiport Switch1/12
  Demux/12 -> Multiport Switch1/13
  Demux/13 -> Multiport Switch1/14
  Demux/14 -> Multiport Switch1/15
  Demux/15 -> Multiport Switch1/16
  Demux/16 -> Multiport Switch1/17
  Demux/17 -> Multiport Switch1/18
  Demux/18 -> Multiport Switch1/19
  Demux/19 -> Multiport Switch1/20
  Demux/20 -> Multiport Switch1/21
  Demux/21 -> Multiport Switch1/22
  Demux/22 -> Multiport Switch1/23
  Demux/23 -> Multiport Switch1/24
  Demux/24 -> Multiport Switch1/25
  Demux/25 -> Multiport Switch1/26
  Demux/26 -> Multiport Switch1/27
  Demux/27 -> Multiport Switch1/28
  Demux/28 -> Multiport Switch1/29
  Demux/29 -> Multiport Switch1/30
  Demux/30 -> Multiport Switch1/31
  From Workspace/1 -> Demux/1
  Demux/31 -> Multiport Switch1/32

== system ModelAgriAuto/Inputs & Data/Weather Inputs/T_a ==
  In1 : Inport
  Gotland 2016 : Constant  Value=|
      | [2.3
      | 5.7
      | 12
      | 15.4
      | 17.7
      | 16.5
      | 14.1
      | 7.5]
  Multiport Switch3 : MultiPortSwitch  Inputs=31  SaturateOnIntegerOverflow=off  InputSameDT=off
  T_a 1989 : Constant  Value=|
      | [2.8
      | 5.2
      | 11.8
      | 15.1
      | 17.3
      | 15.1
      | 12.2
      | 6.9]
  T_a 1990 : Constant  Value=|
      | [4
      | 6.5
      | 11.1
      | 14.4
      | 15.3
      | 16
      | 9.5
      | 6.3]
  T_a 1991 : Constant  Value=|
      | [1.7
      | 5.3
      | 8.1
      | 11.9
      | 17.8
      | 16.5
      | 10.6
      | 6.5]
  T_a 1992 : Constant  Value=|
      | [2.2
      | 2.6
      | 12.9
      | 16.5
      | 16.3
      | 15.2
      | 10.8
      | 2.5]
  T_a 1993 : Constant  Value=|
      | [0.9
      | 5.2
      | 12.6
      | 11.9
      | 16.1
      | 13.2
      | 7.7
      | 4.8]
  T_a 1994 : Constant  Value=|
      | [-0.3
      | 6.2
      | 9
      | 13.2
      | 20
      | 15.6
      | 11
      | 5.3]
  T_a 1995 : Constant  Value=|
      | [1.4
      | 3.4
      | 8.7
      | 15.4
      | 16.8
      | 16.6
      | 11.1
      | 8.4]
  T_a 1996 : Constant  Value=|
      | [-1.7
      | 5.1
      | 7.9
      | 14.3
      | 15.1
      | 17.9
      | 9.2
      | 7.6]
  T_a 1997 : Constant  Value=|
      | [1.6
      | 3.6
      | 8.7
      | 15.6
      | 18.2
      | 19.6
      | 12.1
      | 4.1]
  T_a 1998 : Constant  Value=|
      | [-1.2
      | 3.9
      | 10.1
      | 12.8
      | 15.8
      | 13.7
      | 11.9
      | 5.2]
  T_a 1999 : Constant  Value=|
      | [0.9
      | 6.7
      | 9.4
      | 16.4
      | 18.9
      | 15.1
      | 14.6
      | 7.2]
  T_a 2000 : Constant  Value=|
      | [1.4
      | 6.4
      | 11.9
      | 13.9
      | 15.8
      | 15
      | 10.1
      | 10]
  T_a 2001 : Constant  Value=|
      | [-1.1
      | 5.6
      | 10.7
      | 14.8
      | 19
      | 16.2
      | 11.9
      | 8.8]
  T_a 2002 : Constant  Value=|
      | [1.7
      | 6.5
      | 12
      | 16.6
      | 18.5
      | 19.5
      | 11.9
      | 2.8]
  T_a 2003 : Constant  Value=|
      | [2.7
      | 4.2
      | 11.2
      | 15.4
      | 20.2
      | 16.7
      | 12.5
      | 3.9]
  T_a 2004 : Constant  Value=|
      | [0.9
      | 6.7
      | 10.7
      | 13.9
      | 16.4
      | 17.7
      | 12.8
      | 6.7]
  T_a 2005 : Constant  Value=|
      | [-2.8
      | 6.3
      | 10.4
      | 14.3
      | 18.5
      | 16.1
      | 13
      | 8.1]
  T_a 2006 : Constant  Value=|
      | [-4.1
      | 5.4
      | 10.9
      | 16.7
      | 20
      | 18.4
      | 14.6
      | 8.7]
  T_a 2007 : Constant  Value=|
      | [3.8
      | 7.8
      | 11
      | 16.4
      | 16.9
      | 17.3
      | 11.5
      | 6.8]
  T_a 2008 : Constant  Value=|
      | [0.8
      | 6.3
      | 10.7
      | 15.3
      | 17.3
      | 14.7
      | 10.2
      | 7.1]
  T_a 2009 : Constant  Value=|
      | [-0.1
      | 7.6
      | 11
      | 13
      | 16.8
      | 16.1
      | 12.6
      | 4.1]
  T_a 2010 : Constant  Value=|
      | [-2.4
      | 5.1
      | 10.7
      | 14.5
      | 19.9
      | 16
      | 10.6
      | 4.8]
  T_a 2011 : Constant  Value=|
      | [-0.5
      | 8.3
      | 11.1
      | 16.5
      | 18.1
      | 16.2
      | 13
      | 7.1]
  T_a 2012 : Constant  Value=|
      | [3.4
      | 4.1
      | 10.8
      | 12.8
      | 16.6
      | 15.5
      | 11.4
      | 5.5]
  T_a 2013 : Constant  Value=|
      | [-5
      | 3.7
      | 13.2
      | 15.7
      | 17.1
      | 16.3
      | 11.5
      | 7]
  T_a 2014 : Constant  Value=|
      | [3.5
      | 6.3
      | 10.3
      | 13
      | 19.4
      | 16.3
      | 11.7
      | 8]
  T_a 2015 : Constant  Value=|
      | [2.8
      | 6.3
      | 9.1
      | 13.4
      | 16
      | 16.3
      | 12.2
      | 5.3]
  T_a 2016 : Constant  Value=|
      | [2.2
      | 5.3
      | 11.7
      | 15.1
      | 17.2
      | 15.6
      | 13.7
      | 6.1]
  T_a 2017 : Constant  Value=|
      | [2
      | 3.8
      | 10.2
      | 14.3
      | 16
      | 15.4
      | 12
      | 6.7]
  T_a 2018 : Constant  Value=|
      | [-2.6
      | 6.7
      | 16.1
      | 16.8
      | 22
      | 18.2
      | 13.3
      | 7.7]
  Out1 : Outport  VectorParamsAs1DForOutWhenUnconnected=off
  wires:
  Multiport Switch3/1 -> Out1/1
  In1/1 -> Multiport Switch3/1
  T_a 1994/1 -> Multiport Switch3/7
  T_a 1993/1 -> Multiport Switch3/6
  T_a 1992/1 -> Multiport Switch3/5
  T_a 1991/1 -> Multiport Switch3/4
  T_a 1990/1 -> Multiport Switch3/3
  T_a 1989/1 -> Multiport Switch3/2
  T_a 1995/1 -> Multiport Switch3/8
  T_a 1996/1 -> Multiport Switch3/9
  T_a 1997/1 -> Multiport Switch3/10
  T_a 1998/1 -> Multiport Switch3/11
  T_a 1999/1 -> Multiport Switch3/12
  T_a 2000/1 -> Multiport Switch3/13
  T_a 2001/1 -> Multiport Switch3/14
  T_a 2002/1 -> Multiport Switch3/15
  T_a 2017/1 -> Multiport Switch3/30
  T_a 2016/1 -> Multiport Switch3/29
  T_a 2015/1 -> Multiport Switch3/28
  T_a 2014/1 -> Multiport Switch3/27
  T_a 2013/1 -> Multiport Switch3/26
  T_a 2012/1 -> Multiport Switch3/25
  T_a 2011/1 -> Multiport Switch3/24
  T_a 2010/1 -> Multiport Switch3/23
  T_a 2009/1 -> Multiport Switch3/22
  T_a 2008/1 -> Multiport Switch3/21
  T_a 2018/1 -> Multiport Switch3/31
  T_a 2007/1 -> Multiport Switch3/20
  T_a 2003/1 -> Multiport Switch3/16
  T_a 2004/1 -> Multiport Switch3/17
  T_a 2005/1 -> Multiport Switch3/18
  T_a 2006/1 -> Multiport Switch3/19
  Gotland 2016/1 -> Multiport Switch3/32

== system ModelAgriAuto/Inputs & Data/Weather Inputs/Workability Criterion  ==
  note: X_val==6, byta criteria
  In1 : Inport
  Constant : Constant  Value=6
  Gain2 : Gain  Gain=0.85
  Gain3 : Gain  Gain=1.1
  "I_c =0.75 " : Constant  Value=92.4
  Mueller Trafficability : Constant  Value=69.3
  Multiport Switch : MultiPortSwitch  Inputs=5  DiagnosticForDefault=Warning  SaturateOnIntegerOverflow=off  InputSameDT=off
  Relational Operator : RelationalOperator  Operator===  OutDataTypeStr=boolean  RndMeth=Simplest  InputSameDT=off
  Switch : Switch  Criteria=u2 > Threshold  SaturateOnIntegerOverflow=off  InputSameDT=off
  Out1 : Outport  VectorParamsAs1DForOutWhenUnconnected=off
  wires:
  In1/1 -> Multiport Switch/1
  [PL] -> Multiport Switch/5
  Mueller Trafficability/1 -> Multiport Switch/3
  "I_c =0.75 "/1 -> Multiport Switch/2
  Multiport Switch/1 -> Out1/1
  [X_val] -> Relational Operator/1
  Constant/1 -> Relational Operator/2
  Gain3/1 -> Switch/1
  Gain2/1 -> Switch/3
  Relational Operator/1 -> Switch/2
  Switch/1 -> Multiport Switch/4
  [FC] -> Gain2/1
  [FC] -> Gain3/1
  [FC] -> Multiport Switch/6

== system ModelAgriAuto/Inputs & Data/Weather Inputs/i_h ==
  In1 : Inport
  "Gotland 2016 " : Constant  Value=30.31071421
  I_h 1989 : Constant  Value=28.6394761208436
  I_h 1990 : Constant  Value=26.4369173074403
  I_h 1991 : Constant  Value=25.1362435610033
  I_h 1992 : Constant  Value=26.0301284421133
  I_h 1993 : Constant  Value=21.9986576167445
  I_h 1994 : Constant  Value=26.7241130146822
  I_h 1995 : Constant  Value=26.5924782779521
  I_h 1996 : Constant  Value=25.0470972605219
  I_h 1997 : Constant  Value=28.3314443762401
  I_h 1998 : Constant  Value=22.8804744435833
  I_h 1999 : Constant  Value=30.6117618638391
  I_h 2000 : Constant  Value=28.3184031292242
  I_h 2001 : Constant  Value=29.3897745215641
  I_h 2002 : Constant  Value=30.9495283873874
  I_h 2003 : Constant  Value=29.8279815593933
  I_h 2004 : Constant  Value=28.1633013704692
  I_h 2005 : Constant  Value=29.5789258338055
  I_h 2006 : Constant  Value=34.7860736283004
  I_h 2007 : Constant  Value=30.1566054700424
  I_h 2018 : Constant  Value=37.1486246779653
  Multiport Switch3 : MultiPortSwitch  Inputs=31  SaturateOnIntegerOverflow=off  InputSameDT=off
  i_h 2008 : Constant  Value=26.8953326738992
  i_h 2009 : Constant  Value=27.3620413293233
  i_h 2010 : Constant  Value=27.5337983665195
  i_h 2011 : Constant  Value=31.6381723978199
  i_h 2012 : Constant  Value=25.6932360002149
  i_h 2013 : Constant  Value=29.0353524140376
  i_h 2014 : Constant  Value=29.5680041534911
  i_h 2015 : Constant  Value=26.316972831992
  i_h 2016 : Constant  Value=29.1575102740021
  i_h 2017 : Constant  Value=25.7151344410624
  Out1 : Outport  VectorParamsAs1DForOutWhenUnconnected=off
  wires:
  Multiport Switch3/1 -> Out1/1
  In1/1 -> Multiport Switch3/1
  I_h 2018/1 -> Multiport Switch3/31
  i_h 2017/1 -> Multiport Switch3/30
  i_h 2016/1 -> Multiport Switch3/29
  i_h 2015/1 -> Multiport Switch3/28
  i_h 2014/1 -> Multiport Switch3/27
  i_h 2013/1 -> Multiport Switch3/26
  i_h 2012/1 -> Multiport Switch3/25
  i_h 2011/1 -> Multiport Switch3/24
  i_h 2010/1 -> Multiport Switch3/23
  i_h 2009/1 -> Multiport Switch3/22
  i_h 2008/1 -> Multiport Switch3/21
  I_h 2007/1 -> Multiport Switch3/20
  I_h 2006/1 -> Multiport Switch3/19
  I_h 2005/1 -> Multiport Switch3/18
  I_h 1989/1 -> Multiport Switch3/2
  I_h 1990/1 -> Multiport Switch3/3
  I_h 1991/1 -> Multiport Switch3/4
  I_h 1992/1 -> Multiport Switch3/5
  I_h 1993/1 -> Multiport Switch3/6
  I_h 1994/1 -> Multiport Switch3/7
  I_h 1995/1 -> Multiport Switch3/8
  I_h 1996/1 -> Multiport Switch3/9
  I_h 1997/1 -> Multiport Switch3/10
  I_h 1998/1 -> Multiport Switch3/11
  I_h 1999/1 -> Multiport Switch3/12
  I_h 2000/1 -> Multiport Switch3/13
  I_h 2001/1 -> Multiport Switch3/14
  I_h 2002/1 -> Multiport Switch3/15
  I_h 2003/1 -> Multiport Switch3/16
  I_h 2004/1 -> Multiport Switch3/17
  "Gotland 2016 "/1 -> Multiport Switch3/32

== system ModelAgriAuto/Time & Weather subsyst./Weather & schedule subsystem/Daily soil water content model  ==
  note: Använder Nilsson (2010,2009) och Witney (1988)
  Add : Sum  Inputs=++---
  Constant1 : Constant  Value=0
  Constant4 : Constant  Value=0
  Delay1 : Delay  DelayLength=1  InitialCondition=140
  Integrator : Integrator
  Q r1 : Display
  Q_d (drainage [mm/day]) : Subsystem
  "Q_e (Evotranspiration [mm/day]) " : Subsystem
  "Q_p (precipitation [mm/day]) " : Subsystem
  Q_r (Runoff [mm/day]) : Subsystem
  Scope6 : Scope
  Switch1 : Switch  Criteria=u2 > Threshold  SaturateOnIntegerOverflow=off  InputSameDT=off
  Switch4 : Switch  Criteria=u2 > Threshold  SaturateOnIntegerOverflow=off  InputSameDT=off
  m_a : Display
  m_p (Moisture content previous day [mm]) : Subsystem
  test : Display
  test1 : Display
  m_a (Soil moisture content [mm/m]) : Outport  VectorParamsAs1DForOutWhenUnconnected=off
  tag scope: m_a=global, m_p=global
  wires:
  m_p (Moisture content previous day [mm])/1(Out1) -> [m_p], Q r1/1, Add/1
  Q_r (Runoff [mm/day])/1(Q_r) -> Switch4/2, Switch4/1
  Switch1/1 -> m_a (Soil moisture content [mm/m])/1, m_a/1, [m_a], Delay1/1
  Delay1/1 -> m_p (Moisture content previous day [mm])/1(In1)
  Add/1 -> Switch1/1, Switch1/2
  Constant1/1 -> Switch1/3
  "Q_e (Evotranspiration [mm/day]) "/1(Out1) -> Add/5
  Constant4/1 -> Switch4/3
  Switch4/1 -> Add/3
  Q_d (drainage [mm/day])/1("Q_d ") -> Add/4
  "Q_p (precipitation [mm/day]) "/1(Out1) -> Add/2
  [Q_ph] -> test/1, Scope6/1, "Q_p (precipitation [mm/day]) "/1(In1), Integrator/1
  Integrator/1 -> test1/1

== system ModelAgriAuto/Transport Subsystem/Road forces/Subsystem ==
  a : Inport
  In1 : Inport  Port=2
  Add : Sum
  Constant : Constant  Value=1/60
  Constant1 : Constant  Value=2
  Display : Display
  F_a_road : Product
  Gain : Gain  Gain=1/1000
  Product : Product  Inputs=3
  Product1 : Product
  Product2 : Product
  tag scope: E_a=global
  wires:
  F_a_road/1 -> Add/1
  [m] -> F_a_road/1
  a/1 -> F_a_road/2
  [F_road] -> Add/2
  Add/1 -> Product/1
  [v_road] -> Product/2
  Constant/1 -> Product/3
  In1/1 -> Product1/2
  Constant1/1 -> Product1/1
  Product2/1 -> Gain/1
  Product1/1 -> Product2/2
  Product/1 -> Product2/1
  Gain/1 -> [E_a], Display/1

== system ModelAgriAuto/Inputs & Data/Battery and driveline inputs/Battery capacity reduction/Charging rate choice ==
  note: 0.1c
  note: 1c
  note: 4c
  note: 0.1c
  Constant : Constant  Value=-8.81e-13
  Constant1 : Constant  Value=7.65e-9
  Constant10 : Constant  Value=-1.69e-4
  Constant11 : Constant  Value=0.9371
  Constant12 : Constant  Value=C_rate
  Constant2 : Constant  Value=-2.97e-5
  Constant3 : Constant  Value=0.9820
  Constant4 : Constant  Value=-3.37e-12
  Constant5 : Constant  Value=2.77e-8
  Constant6 : Constant  Value=-9.6e-5
  Constant7 : Constant  Value=0.9655
  Constant8 : Constant  Value=-7.07e-12
  Constant9 : Constant  Value=5.43e-8
  Demux : Demux
  Multiport Switch : MultiPortSwitch  DataPortForDefault=Additional data port  SaturateOnIntegerOverflow=off  InputSameDT=off
  Mux : Mux
  Mux1 : Mux
  Mux2 : Mux
  Out1 : Outport
  Out2 : Outport  Port=2
  Out3 : Outport  Port=3
  Out4 : Outport  Port=4
  wires:
  Constant/1 -> Mux/1
  Constant1/1 -> Mux/2
  Constant2/1 -> Mux/3
  Constant3/1 -> Mux/4
  Constant7/1 -> Mux1/4
  Constant4/1 -> Mux1/1
  Constant6/1 -> Mux1/3
  Constant5/1 -> Mux1/2
  Constant11/1 -> Mux2/4
  Constant8/1 -> Mux2/1
  Constant10/1 -> Mux2/3
  Constant9/1 -> Mux2/2
  Demux/1 -> Out1/1  "a"
  Demux/2 -> Out2/1  "b"
  Demux/3 -> Out3/1  "c"
  Demux/4 -> Out4/1  "d"
  Multiport Switch/1 -> Demux/1
  Mux2/1 -> Multiport Switch/4
  Mux1/1 -> Multiport Switch/5, Multiport Switch/3
  Mux/1 -> Multiport Switch/2
  Constant12/1 -> Multiport Switch/1

== system ModelAgriAuto/Inputs & Data/Field inputs/Field forces/Acceleration force calculator ==
  In1 : Inport
  MATLAB Function : MATLAB Function  TreatAsAtomicUnit=on
  Out1 : Outport  VectorParamsAs1DForOutWhenUnconnected=off
  wires:
  In1/1 -> MATLAB Function/1(a)
  MATLAB Function/1(F_a_field) -> Out1/1

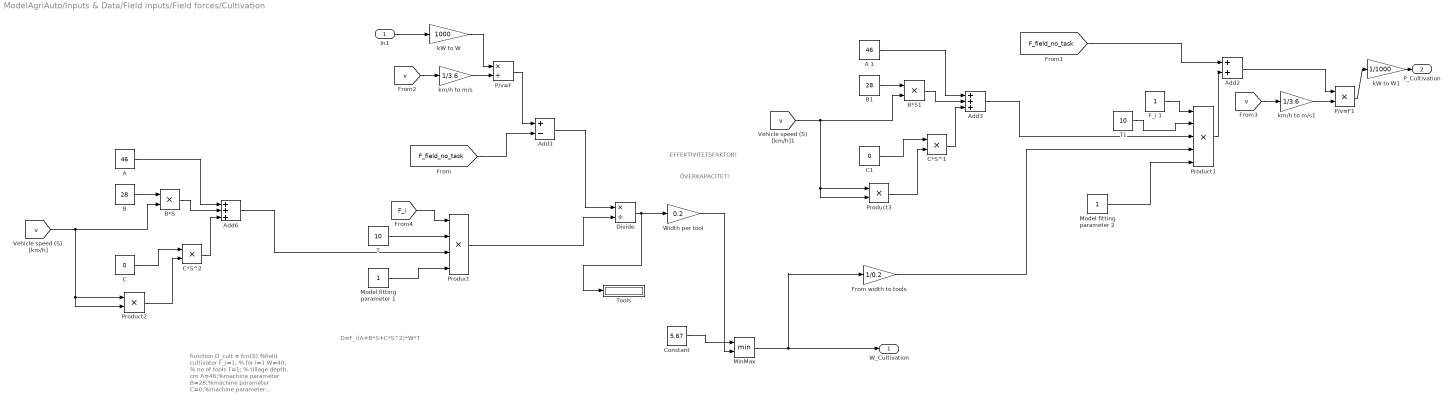
== system ModelAgriAuto/Inputs & Data/Field inputs/Field forces/Cultivation ==
  note: function D_cult = fcn(S)
      |
      | %field cultivator
      |
      | F_i=1; % for i=1
      | W=40; % no of tools
      | T=1; % tillage depth, cm
      | A=46;%machine parameter
      | B=28;%machine parameter
      | C=0;%machine parameter
      |
      | D_cult=F_i*(A+B*S+C*S^2)*W*T;
  note: D=F_i(A+B*S+C*S^2)*W*T
  note: ÖVERKAPACITET!
  note: EFFEKTIVITETSFAKTOR!
  In1 : Inport
  "A " : Constant  Value=46
  A 1 : Constant  Value=46
  Add1 : Sum  Inputs=+-
  Add2 : Sum
  Add3 : Sum  Inputs=+++
  Add6 : Sum  Inputs=+++
  B : Constant  Value=28
  B*S : Product
  B*S1 : Product
  B1 : Constant  Value=28
  C : Constant  Value=0
  C*S^1 : Product
  C*S^2 : Product
  C1 : Constant  Value=0
  Constant : Constant  Value=5.67
  Divide : Product  Inputs=*/
  F_i 1 : Constant
  "From width to tools " : Gain  Gain=1/0.2
  MinMax : MinMax  Inputs=2
  Model fitting parameter 1 : Constant
  Model fitting parameter 2 : Constant
  P/v=F : Product  Inputs=*/
  P/v=F1 : Product  Inputs=**
  Product : Product  Inputs=4
  Product1 : Product  Inputs=5
  Product2 : Product
  Product3 : Product
  T : Constant  Value=10
  T1 : Constant  Value=10
  Tools : Display
  Width per tool : Gain  Gain=0.2
  kW to W : Gain  Gain=1000
  kW to W1 : Gain  Gain=1/1000
  km/h to m/s : Gain  Gain=1/3.6
  km/h to m/s1 : Gain  Gain=1/3.6
  W_Cultivation : Outport  VectorParamsAs1DForOutWhenUnconnected=off
  P_Cultivation : Outport  Port=2  VectorParamsAs1DForOutWhenUnconnected=off
  wires:
  "A "/1 -> Add6/1
  B/1 -> B*S/1
  [v] -> km/h to m/s/1
  B*S/1 -> Add6/2
  Add6/1 -> Product/3
  Product/1 -> Divide/2
  [F_i] -> Product/1
  Divide/1 -> Tools/1, Width per tool/1
  C/1 -> C*S^2/1
  kW to W/1 -> P/v=F/1
  km/h to m/s/1 -> P/v=F/2
  [F_field_no_task] -> Add1/2
  Add1/1 -> Divide/1
  [v] -> Product2/2, Product2/1, B*S/2
  In1/1 -> kW to W/1
  Product2/1 -> C*S^2/2
  C*S^2/1 -> Add6/3
  T/1 -> Product/2
  Width per tool/1 -> MinMax/2
  Constant/1 -> MinMax/1
  P/v=F/1 -> Add1/1
  MinMax/1 -> "From width to tools "/1, W_Cultivation/1
  A 1/1 -> Add3/1
  T1/1 -> Product1/2
  C1/1 -> C*S^1/1
  Product3/1 -> C*S^1/2
  Add2/1 -> P/v=F1/1
  kW to W1/1 -> P_Cultivation/1
  Product1/1 -> Add2/2
  Add3/1 -> Product1/3
  [v] -> Product3/2, Product3/1, B*S1/2
  B*S1/1 -> Add3/2
  [F_field_no_task] -> Add2/1
  B1/1 -> B*S1/1
  F_i 1/1 -> Product1/1
  C*S^1/1 -> Add3/3
  Model fitting parameter 1/1 -> Product/4
  Model fitting parameter 2/1 -> Product1/5
  "From width to tools "/1 -> Product1/4
  [v] -> km/h to m/s1/1
  km/h to m/s1/1 -> P/v=F1/2
  P/v=F1/1 -> kW to W1/1

== system ModelAgriAuto/Inputs & Data/Field inputs/Field forces/Drag force calculator ==
  v_field : Inport
  MATLAB Function : MATLAB Function  TreatAsAtomicUnit=on
  F_drag_field : Outport  VectorParamsAs1DForOutWhenUnconnected=off
  wires:
  v_field/1 -> MATLAB Function/1(v)
  MATLAB Function/1(F_drag_field) -> F_drag_field/1

== system ModelAgriAuto/Inputs & Data/Field inputs/Field forces/Fert Spreading ==
  note: EMMA och Engström/Lagnelöv 2017
  In2 : Inport
  Add : Sum  Inputs=+-
  Add4 : Sum
  Constant1 : Constant  Commented=on  Value=3.1159
  Constant2 : Constant  Commented=on  Value=2.33
  F*v=P : Product  Inputs=**
  MinMax : MinMax  Inputs=2
  "P spread \"fastgödsel\" [kW]" : Constant  Commented=on  Value=48
  "P spread \"kletgödsel\" [kW]" : Constant  Commented=on  Value=43
  "P spread \"konstgödsel\" [kW]" : Constant  Commented=on  Value=16
  "P spread \"urin\" [kW] " : Constant  Commented=on  Value=28
  P/(P/w)=w : Product  Inputs=*/
  P/(P/w)=w1 : Product  Inputs=**
  P/v=F2 : Product  Inputs=**
  "W spread \"art. fert.\" [m]" : Constant  Value=24
  "W spread \"fastgödsel\" [m]" : Constant  Commented=on  Value=6
  "W spread \"kletgödsel\" [m]1" : Constant  Commented=on  Value=13.8
  "W spread \"konstgödsel\" [m]" : Constant  Commented=on  Value=22
  "W spread \"urin\" [m]" : Constant  Commented=on  Value=12
  W_display1 : Display
  "ha/h \"kletgödsel\" " : Constant  Commented=on  Value=6.9
  "ha/h \"konstgödsel\" " : Constant  Commented=on  Value=11
  kW to W1 : Gain  Gain=1/1000
  kW to W3 : Gain  Gain=1/1000
  kW/m : Constant  Commented=on  Value=0.7273
  "kW/m \"kletgödsel\" [kW/m] " : Constant  Value=3.1159
  km/h to m/s1 : Gain  Gain=1/3.6
  km/h to m/s3 : Gain  Gain=1/3.6
  kw/m : Constant  Commented=on  Value=8
  W_spread : Outport  VectorParamsAs1DForOutWhenUnconnected=off
  P_spread : Outport  Port=2  VectorParamsAs1DForOutWhenUnconnected=off
  wires:
  In2/1 -> Add/1
  [F_field_no_task] -> kW to W1/1
  MinMax/1 -> P/(P/w)=w1/1, W_spread/1
  "W spread \"art. fert.\" [m]"/1 -> MinMax/1
  kW to W1/1 -> F*v=P/1
  [v] -> km/h to m/s1/1
  km/h to m/s1/1 -> F*v=P/2
  F*v=P/1 -> Add/2
  Add/1 -> W_display1/1, P/(P/w)=w/1
  "kW/m \"kletgödsel\" [kW/m] "/1 -> P/(P/w)=w1/2, P/(P/w)=w/2
  P/(P/w)=w/1 -> MinMax/2
  P/(P/w)=w1/1 -> Add4/2
  km/h to m/s3/1 -> P/v=F2/2
  [F_field_no_task] -> P/v=F2/1
  kW to W3/1 -> Add4/1
  [v] -> km/h to m/s3/1
  P/v=F2/1 -> kW to W3/1
  Add4/1 -> P_spread/1

== system ModelAgriAuto/Inputs & Data/Field inputs/Field forces/Gradient force calculator1 ==
  grad : Inport
  MATLAB Function : MATLAB Function  TreatAsAtomicUnit=on
  F_grad_field : Outport  VectorParamsAs1DForOutWhenUnconnected=off
  wires:
  grad/1 -> MATLAB Function/1(grad)
  MATLAB Function/1(F_grad_field) -> F_grad_field/1
